simulink model "feedbackLineariz2"  (Simulink 7.7)
settings: Solver=FixedStepDiscrete  StartTime=0.0  StopTime=Inf  FixedStep=Ts  RelTol=1e-3
PreLoadFcn:
  | initFeedLin;
InitFcn:
  | initFeedLin;
values from neighbouring files (symbols this model uses):
  gains = [50*kp,ki*10,kd*7]    [initFeedLin.m]
  qDes = [ 1.1695 ... (first row only)    [initFeedLin.m]
  Ts = 0.01    [initFeedLin.m]
undefined symbols (not defined in the file or in its folder): DiscIntNeverNeededParam
libraries: WBCLibrary x7, utility x1
settings Model: Creator=iron  LastModifiedBy=iron

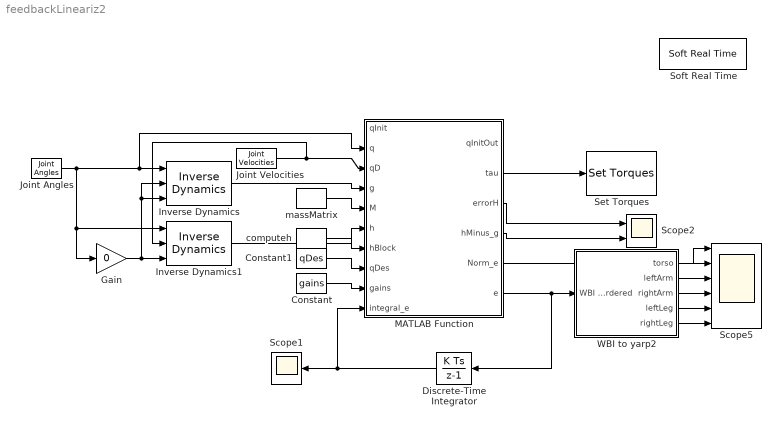
== system feedbackLineariz2 ==
  Constant : Constant  Value=gains
  Constant1 : Constant  Value=qDes
  Discrete-Time Integrator : DiscreteIntegrator  InitialCondition=zeros(25,1)  SampleTime=Ts  ICPrevOutput=DiscIntNeverNeededParam  ICPrevScaledInput=DiscIntNeverNeededParam
  Gain : Gain  Gain=0
  Inverse Dynamics : WBCLibrary/wholeBodyModel/Dynamics/Inverse Dynamics  SystemSampleTime=-1  robotName=robotName  localName=localName
  Inverse Dynamics1 : WBCLibrary/wholeBodyModel/Dynamics/Inverse Dynamics  SystemSampleTime=-1  robotName=robotName  localName=localName
  Joint Angles : WBCLibrary/wholeBodyStates/Joint Angles  SystemSampleTime=-1  robotName=robotName  localName=localName
  Joint Velocities : WBCLibrary/wholeBodyStates/Joint Velocities  SystemSampleTime=-1  robotName=robotName  localName=localName
  MATLAB Function : Stateflow chart  TreatAsAtomicUnit=on
  Scope1 : Scope
      settings: YMin=-1  YMax=1.5
  Scope2 : Scope  NumInputPorts=2
      settings: YMin=0~-1  YMax=8.5e-17~1
  Scope5 : Scope  NumInputPorts=6
      settings: TimeRange=18  YMin=50~-0.75~-0.75~-1~-1~-1.5  YMax=170~1.5~0.75~1~1~1.25  SaveName=ScopeData2
  Set Torques : WBCLibrary/wholeBodyActuators/Set Torques  SystemSampleTime=-1  val=6  robotName=robotName  localName=localName
  Soft Real Time : utility/Soft Real Time  x=Ts
  WBI to yarp2 : Subsystem
  computeh : WBCLibrary/wholeBodyModel/Dynamics/computeh  SystemSampleTime=-1  val=7  robotname=robotName  localname=localName
  massMatrix : WBCLibrary/wholeBodyModel/Dynamics/massMatrix  SystemSampleTime=-1  val=8  robotname=robotName  localname=localName
  wires:
  Joint Angles/1 -> Inverse Dynamics1/1, Gain/1, Inverse Dynamics/1, MATLAB Function/2(q)
  Gain/1 -> Inverse Dynamics/2, Inverse Dynamics/3, Inverse Dynamics1/3
  Joint Velocities/1 -> Inverse Dynamics1/2, MATLAB Function/3(qD)
  Inverse Dynamics/1 -> MATLAB Function/4(g)
  massMatrix/1 -> MATLAB Function/5(M)
  Inverse Dynamics1/1 -> MATLAB Function/6(h)
  MATLAB Function/6(e) -> WBI to yarp2/1(WBI ordered), Discrete-Time Integrator/1
  Constant1/1 -> MATLAB Function/8(qDes)
  Discrete-Time Integrator/1 -> Scope1/1, MATLAB Function/10(integral_e)
  Constant/1 -> MATLAB Function/9(gains)
  WBI to yarp2/5(rightLeg) -> Scope5/6
  WBI to yarp2/4(leftLeg) -> Scope5/5
  WBI to yarp2/3(rightArm) -> Scope5/4
  WBI to yarp2/2(leftArm) -> Scope5/3
  WBI to yarp2/1(torso) -> Scope5/2
  MATLAB Function/5(Norm_e) -> Scope5/1
  computeh/1 -> MATLAB Function/7(hBlock)
  MATLAB Function/3(errorH) -> Scope2/1
  MATLAB Function/4(hMinus_g) -> Scope2/2
  MATLAB Function/2(tau) -> Set Torques/1

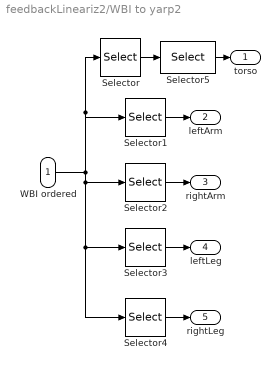
== system feedbackLineariz2/WBI to yarp2 ==
  WBI ordered : Inport
  Selector : Selector  InputPortWidth=25  IndexOptions=Index vector (dialog)  Indices=[1 2 3]  OutputSizes=1
  Selector1 : Selector  InputPortWidth=25  IndexOptions=Index vector (dialog)  Indices=[4 5 6 7 8]  OutputSizes=1
  Selector2 : Selector  InputPortWidth=25  IndexOptions=Index vector (dialog)  Indices=[9 10 11 12 13]  OutputSizes=1
  Selector3 : Selector  InputPortWidth=25  IndexOptions=Index vector (dialog)  Indices=[14 15 16 17 18 19]  OutputSizes=1
  Selector4 : Selector  InputPortWidth=25  IndexOptions=Index vector (dialog)  Indices=[20 21 22 23 24 25]  OutputSizes=1
  Selector5 : Selector  InputPortWidth=3  IndexOptions=Index vector (dialog)  Indices=[3 2 1]  OutputSizes=1
  torso : Outport
  leftArm : Outport  Port=2
  rightArm : Outport  Port=3
  leftLeg : Outport  Port=4
  rightLeg : Outport  Port=5
  wires:
  Selector1/1 -> leftArm/1
  Selector2/1 -> rightArm/1
  Selector3/1 -> leftLeg/1
  Selector4/1 -> rightLeg/1
  WBI ordered/1 -> Selector/1, Selector1/1, Selector2/1, Selector4/1, Selector3/1
  Selector/1 -> Selector5/1
  Selector5/1 -> torso/1

== matlab function MATLAB Function ==
  data: qInit input double; qInitOut output double; q input double; qD input double; g input double; M input double; h input double; hBlock input double; qDes input double; gains input double; integral_e input double; tau output double; errorH output double; hMinus_g output double; Norm_e output double; e output double
function [qInitOut,tau,errorH,hMinus_g,Norm_e,e] = fcn(qInit,q,qD,g,M,h,hBlock,qDes,gains,integral_e)
%#codegen

qInitOut = qInit;

e = q-qDes;

Norm_e = norm(e)*180/pi;

kp = gains(:,1:25);
ki = gains(:,26:50);
kd = gains(:,51:75);

tau = g - (kp*e + ki*integral_e + kd*qD);

errorH = h - hBlock(7:end);

hMinus_g = h - g;

tau = tau*0;
